simulink model "test1"  (R2021b)
settings: Solver=FixedStepAuto  StartTime=0.0  StopTime=10.0  RelTol=1e-3
libraries: arduinolib x2, simulink x1, arduinosensorlib x1, arduinomotorcarrierlib x1
settings Model: ExtModeTrigDuration=2  Creator=cwpan  LastModifiedBy=cwpan
settings OptimizationCC: EnhancedBackFolding=on  PassReuseOutputArgsAs=Individual arguments  ZeroExternalMemoryAtStartup=off  ZeroInternalMemoryAtStartup=off  MaxStackSize=64  OptimizeBlockOrder=speed  DifferentSizesBufferReuse=on  OptimizationCustomize=off  EfficientTunableParamExpr=on
settings DebuggingCC: ParameterTunabilityLossMsg=error
settings HardwareCC: ProdBitPerPointer=32  ProdBitPerSizeT=32  ProdBitPerPtrDiffT=32  ProdLargestAtomicInteger=Long  ProdLargestAtomicFloat=Double  ProdWordSize=32  ProdHWDeviceType=ARM Compatible->ARM Cortex  UseEmbeddedCoderFeatures=off  UseSimulinkCoderFeatures=off
settings SFSimCC: MATLABDynamicMemAlloc=off
settings RTWCC: Description=Embedded Coder  SystemTargetFile=ert.tlc  HardwareBoard=Arduino Nano 33 BLE Sense  TemplateMakefile=ert_default_tmf  Toolchain=Arduino ARM MBED  BuildConfiguration=Faster Runs
settings CodeAppCC: ForceParamTrailComments=on  IgnoreCustomStorageClasses=off  OperatorAnnotations=on  SimulinkDataObjDesc=on  SFDataObjDesc=on  InsertBlockDesc=on
settings ERTTargetCC: SupportContinuousTime=on  SupportNonInlinedSFcns=on  SupportVariableSizeSignals=on  ExtModeTransport=3  ExtModeStaticAlloc=on  ExtModeStaticAllocSize=65536  ExtModeMexFile=ext_xcp  ExtModeIntrfLevel=Level2 - Open

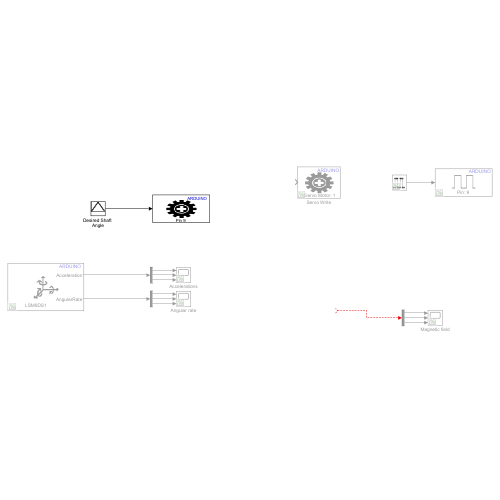
[thumbnail: Simulink's stored preview of the top-level diagram]
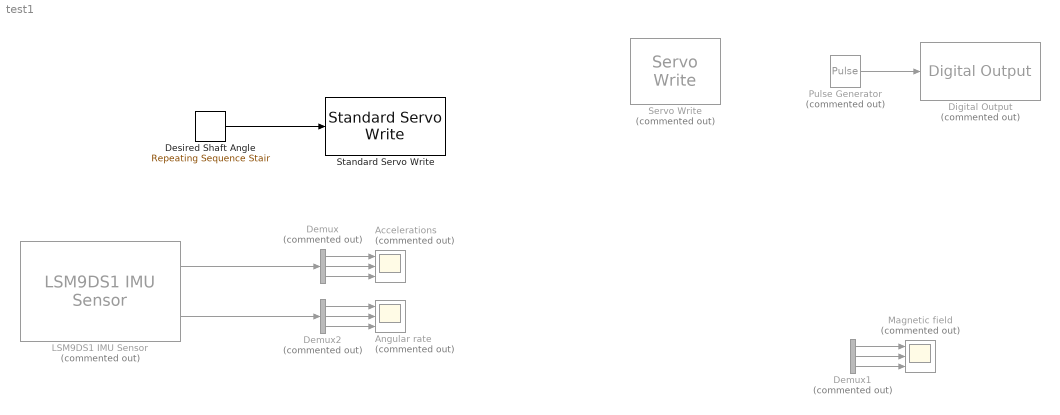
== system test1 ==
  Accelerations : Scope  Commented=on  NumInputPorts=3
  Angular rate : Scope  Commented=on  NumInputPorts=3
  Demux : Demux  Commented=on  Outputs=3
  Demux1 : Demux  Commented=on  Outputs=3
  Demux2 : Demux  Commented=on  Outputs=3
  Desired Shaft Angle : simulink/Sources/Repeating Sequence Stair  OutValues=[0:180 179:-1:1]  tsamp=0.01  OutMin=[]  OutMax=[]  OutDataTypeStr=uint8  OutputDataTypeScalingMode=uint8  OutDataType=fixdt(0,8)  ConRadixGroup=Best Precision: Vector-wise  OutScaling=2^-12
  Digital Output : arduinolib/Digital Output  Commented=on  pinNumber=9  Direction=output  blockPlatform=arduino
  LSM9DS1 IMU Sensor : arduinosensorlib/LSM9DS1 IMU Sensor  Commented=on  AccelandGyroAddress=0x6A  MagnetometerAddress=0x1C  EnableAccel=on  EnableGyro=on  EnableMag=off  AccelerometerOutputDataRate=119 Hz  AccelerometerFullScaleRange=+/- 2g  AccelerometerBandwidth=50 Hz  GyroscopeOutputDataRate=119 Hz  GyroscopeFullScaleRange=245 dps  GyroscopeBandwidthMode=0  GyroscopeHighPassFilterEnabled=on  GyroscopeHighPassFilterMode=0  MagnetometerOutputDataRate=40 Hz  MagnetometerFullScaleRange=+/- 4 gauss  SampleTime=0.1
      settings: SourceProductBaseCode=ARDUINO
  Magnetic field : Scope  Commented=on  NumInputPorts=3
  Pulse Generator : DiscretePulseGenerator  Commented=on  Period=10  PulseWidth=5  SampleTime=0.1
  Servo Write : arduinomotorcarrierlib/Servo Write  Commented=on  SlaveAddress=uint8( hex2dec( '66' ) )  blockPlatform=ARDUINO  MotorNumber=1  MotorCarrierPWMFreq=100
      settings: SourceProductBaseCode=ARDUINO
  Standard Servo Write : arduinolib/Standard Servo Write  pinNumber=9  ServoIndex=0  blockPlatform=ARDUINO
  wires:
  Pulse Generator/1 -> Digital Output/1
  LSM9DS1 IMU Sensor/1 -> Demux/1
  LSM9DS1 IMU Sensor/2 -> Demux2/1
  Demux/1 -> Accelerations/1
  Demux/2 -> Accelerations/2
  Demux/3 -> Accelerations/3
  Demux2/1 -> Angular rate/1
  Demux2/2 -> Angular rate/2
  Demux2/3 -> Angular rate/3
  Demux1/1 -> Magnetic field/1
  Demux1/3 -> Magnetic field/3
  ? -> Demux1/1
  Demux1/2 -> Magnetic field/2
  Desired Shaft Angle/1 -> Standard Servo Write/1
